simulink model "Regler_fin"  (R2026a)
settings: Solver=ode23s  StartTime=tSim(1)  StopTime=tSim(end)  FixedStep=tStep  EnableMultiTasking=on
values from neighbouring files (symbols this model uses):
  A_grid = zeros(N_ml, 16)    [reglerInit_fin.m]    (also in reglerInit_opt1.m; reglerInit_opt2.m; reglerInit_opt3.m; reglerInit_opt4.m)
  a_ref0 = 0    [reglerInit_fin.m]    (also in reglerInit_opt2.m; reglerInit_opt3.m; reglerInit_opt4.m)
  a_ref_lim = 3.91175    [reglerInit_fin.m]    (also in reglerInit_opt2.m = 3.8; reglerInit_opt3.m = 3.8)
  B = [0; -30.49; 0; 30.49]    [A4_4.m]    (also in reglerInit.m; reglerInit_fin.m; reglerInit_gain_scheduling.m; reglerInit_opt.m)
  C = [1 0 0 0 ... (first row only)    [reglerInit.m]    (also in reglerInit_fin.m; reglerInit_gain_scheduling.m; reglerInit_opt.m; reglerInit_opt1.m)
  d_large = 1.18779    [reglerInit_fin.m]    (also in reglerInit_opt2.m = 1.3; reglerInit_opt3.m = 1.3; reglerInit_opt4.m = 1.2)
  d_small = 0.5719    [reglerInit_fin.m]    (also in reglerInit_opt2.m = 0.45; reglerInit_opt3.m = 0.45; reglerInit_opt4.m = 0.35)
  ff_gain = 0.942931    [reglerInit_fin.m]    (also in reglerInit_opt.m = 1; reglerInit_opt1.m = 1; reglerInit_opt2.m = 1; reglerInit_opt3.m = 1)
  g = 9.81    [reglerInit_fin.m]    (also in reglerInit_opt.m; reglerInit_opt1.m; reglerInit_opt2.m; reglerInit_opt3.m)
  gamma_phi = 0.195386    [reglerInit_fin.m]    (also in reglerInit_opt2.m = 0.3; reglerInit_opt3.m = 0.3; reglerInit_opt4.m = 0)
  j_ref_lim = 24.6332    [reglerInit_fin.m]    (also in reglerInit_opt2.m = 20; reglerInit_opt3.m = 20)
  K_grid = zeros(N_ml, 4)    [reglerInit_fin.m]    (also in reglerInit_opt1.m; reglerInit_opt2.m)
  k_r = 7.2e-3    (= 0.0072)    [reglerInit_fin.m]    (also in reglerInit_opt.m; reglerInit_opt1.m; reglerInit_opt2.m; reglerInit_opt3.m)
  L_grid = zeros(N_ml, 8)    [reglerInit_fin.m]    (also in reglerInit_opt1.m; reglerInit_opt2.m; reglerInit_opt3.m; reglerInit_opt4.m)
  M_ff_max = 0.39    [reglerInit_fin.m]    (also in reglerInit_opt.m = 0.34; reglerInit_opt1.m = 0.34; reglerInit_opt2.m = 0.34; reglerInit_opt3.m = 0.34)
  M_max_total = 0.4    [reglerInit.m]    (also in reglerInit_fin.m; reglerInit_gain_scheduling.m; reglerInit_opt.m; reglerInit_opt1.m)
  m_s = 0.8    [reglerInit_fin.m]    (also in reglerInit_opt.m; reglerInit_opt1.m; reglerInit_opt2.m; reglerInit_opt3.m)
  ml_grid = linspace(1, 5, 17)    [reglerInit_fin.m]    (also in reglerInit_opt1.m; reglerInit_opt2.m; reglerInit_opt3.m; reglerInit_opt4.m)
  omega_ref_large = 2.08014    [reglerInit_fin.m]    (also in reglerInit_opt2.m = 2; reglerInit_opt3.m = 2)
  omega_ref_medium = 3.57058    [reglerInit_fin.m]    (also in reglerInit_opt2.m = 3.3; reglerInit_opt3.m = 3.3)
  omega_ref_small = 3.92272    [reglerInit_fin.m]    (also in reglerInit_opt2.m = 3.3; reglerInit_opt3.m = 3.3)
  phi_ref_lim = deg2rad(35)    [reglerInit_fin.m]    (also in reglerInit_opt2.m = deg2rad(18); reglerInit_opt3.m = deg2rad(18); reglerInit_opt4.m = deg2rad(10))
  phi_slow_1 = deg2rad(26.517)    [reglerInit_fin.m]    (also in reglerInit_opt2.m = deg2rad(28); reglerInit_opt3.m = deg2rad(28); reglerInit_opt4.m = deg2rad(28))
  phi_slow_2 = deg2rad(30.8674)    [reglerInit_fin.m]    (also in reglerInit_opt2.m = deg2rad(36); reglerInit_opt3.m = deg2rad(36); reglerInit_opt4.m = deg2rad(36))
  phidot_ref_lim = 1.6    [reglerInit_fin.m]    (also in reglerInit_opt2.m = 0.8; reglerInit_opt3.m = 0.8; reglerInit_opt4.m = 0)
  r_wheel = 0.041    [reglerInit_fin.m]    (also in reglerInit_opt.m; reglerInit_opt1.m; reglerInit_opt2.m; reglerInit_opt3.m)
  u_max = 100    [reglerInit.m]    (also in reglerInit_fin.m; reglerInit_gain_scheduling.m; reglerInit_opt.m; reglerInit_opt1.m)
  v_ref0 = 0    [reglerInit_fin.m]    (also in reglerInit_opt2.m; reglerInit_opt3.m; reglerInit_opt4.m)
  x_ref0 = 0    [reglerInit_fin.m]    (also in reglerInit_opt2.m; reglerInit_opt3.m; reglerInit_opt4.m)
  xhat0 = [0, 0, 0, 0]    [reglerInit.m]    (also in reglerInit_fin.m = [0; 0; 0; 0]; reglerInit_gain_scheduling.m; reglerInit_opt.m = [0; 0; 0; 0]; reglerInit_opt1.m = [0; 0; 0; 0])
settings Model: Creator=Henning Schlüter  LastModifiedBy=louis
settings DataIOCC: SignalLoggingSaveFormat=ModelDataLogs
settings DebuggingCC: UnderspecifiedInitializationDetection=Classic  PregeneratedLibrarySubsystemCodeDiagnostic=none
settings HardwareCC: ProdHWDeviceType=32-bit Generic
settings GRTTargetCC: CombineOutputUpdateFcns=off  GRTInterface=on

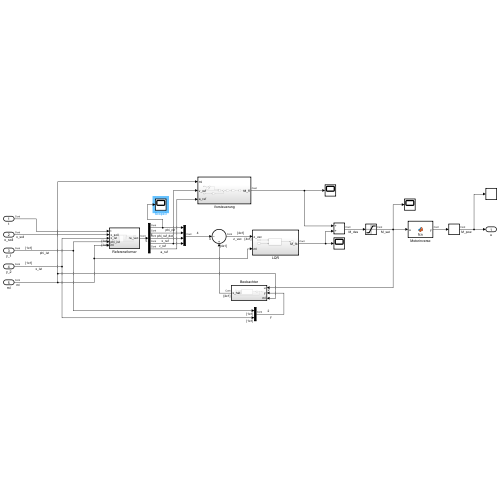
[thumbnail: Simulink's stored preview of the top-level diagram]
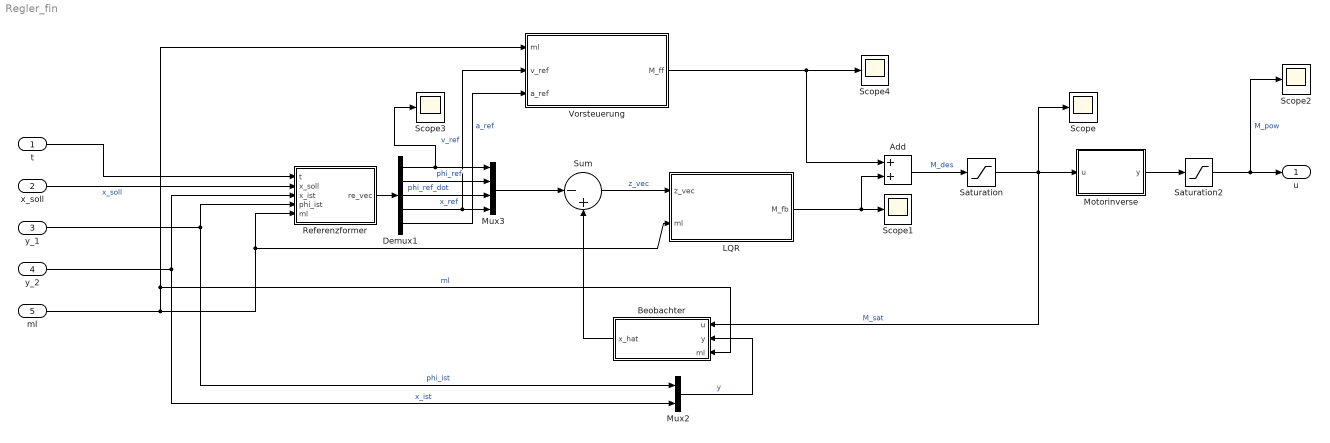
== system Regler_fin ==
  t : Inport  OutDataTypeStr=double  PortDimensions=1  SampleTime=0
  "x_soll " : Inport  Port=2  OutDataTypeStr=double  PortDimensions=1  SampleTime=0
  y_1 : Inport  Port=3  OutDataTypeStr=double  PortDimensions=[1 1]  SampleTime=0
  y_2 : Inport  Port=4  OutDataTypeStr=double  PortDimensions=[1 1]  SampleTime=0
  ml : Inport  Port=5  OutDataTypeStr=double  PortDimensions=1  SampleTime=0
  Add : Sum
  Beobachter : Subsystem
  Demux1 : Demux  Outputs=5
  LQR : Subsystem
  Motorinverse : MATLAB Function  TreatAsAtomicUnit=on
  Mux2 : Mux  Inputs=2
  Mux3 : Mux
  Referenzformer : Subsystem
  Saturation : Saturate  UpperLimit=M_max_total  LowerLimit=-M_max_total
  Saturation2 : Saturate  UpperLimit=u_max  LowerLimit=-u_max  LinearizeAsGain=off
  Scope{,1..4} (5 alike) : Scope
      Scope settings: ActiveDisplayYMinimum=-0.49175375586070769  ActiveDisplayYMaximum=-0.20102751095454277
      Scope1 settings: ActiveDisplayYMinimum=-0.094687281937852363  ActiveDisplayYMaximum=1.6990664417619266
      Scope2 settings: ActiveDisplayYMinimum=27.519723000110169  ActiveDisplayYMaximum=88.458122086201712  DataLoggingVariableName=ScopeData2
      Scope3 settings: ActiveDisplayYMinimum=-0.061908248725805554  ActiveDisplayYMaximum=0.071206311299841979  DataLoggingVariableName=ScopeData3
      Scope4 settings: ActiveDisplayYMinimum=-0.15043823578049448  ActiveDisplayYMaximum=0.16991782466155569  DataLoggingVariableName=ScopeData6
  Sum : Sum  Inputs=|-+
  Vorsteuerung : Subsystem
  u : Outport  OutDataTypeStr=double  PortDimensions=1  VectorParamsAs1DForOutWhenUnconnected=off
  wires:
  Saturation/1 -> Motorinverse/1(u), Beobachter/1(u), Scope/1  "M_sat"
  Motorinverse/1(y) -> Saturation2/1
  Referenzformer/1(re_vec) -> Demux1/1
  y_2/1 -> Mux2/2, Referenzformer/3(x_ist)  "x_ist"
  Saturation2/1 -> u/1, Scope2/1  "M_pow"
  t/1 -> Referenzformer/1(t)
  Mux2/1 -> Beobachter/2(y)  "y"
  "x_soll "/1 -> Referenzformer/2(x_soll)  "x_soll"
  y_1/1 -> Referenzformer/4(phi_ist), Mux2/1  "phi_ist"
  ml/1 -> Beobachter/3(ml), Vorsteuerung/1(ml), LQR/2(ml), Referenzformer/5(ml)  "ml"
  Demux1/1 -> Scope3/1, Mux3/1  "phi_ref"
  Demux1/2 -> Mux3/2  "phi_ref_dot"
  Demux1/3 -> Mux3/3  "x_ref"
  Demux1/4 -> Mux3/4, Vorsteuerung/2(v_ref)  "v_ref"
  Mux3/1 -> Sum/1
  Add/1 -> Saturation/1  "M_des"
  Demux1/5 -> Vorsteuerung/3(a_ref)  "a_ref"
  LQR/1(M_fb) -> Add/2, Scope1/1
  Sum/1 -> LQR/1(z_vec)  "z_vec"
  Beobachter/1(x_hat) -> Sum/2
  Vorsteuerung/1(M_ff) -> Add/1, Scope4/1

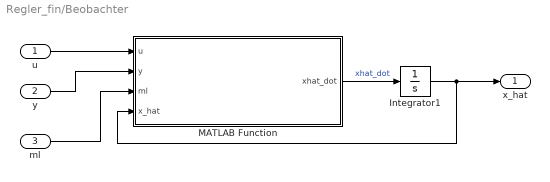
== system Regler_fin/Beobachter ==
  u : Inport
  y : Inport  Port=2
  ml : Inport  Port=3
  Integrator1 : Integrator  InitialCondition=xhat0
  MATLAB Function : MATLAB Function  TreatAsAtomicUnit=on
  x_hat : Outport
  wires:
  u/1 -> MATLAB Function/1(u)
  MATLAB Function/1(xhat_dot) -> Integrator1/1  "xhat_dot"
  Integrator1/1 -> MATLAB Function/4(x_hat), x_hat/1
  ml/1 -> MATLAB Function/3(ml)
  y/1 -> MATLAB Function/2(y)

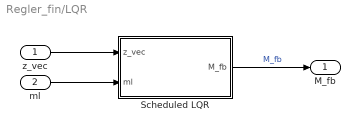
== system Regler_fin/LQR ==
  z_vec : Inport
  ml : Inport  Port=2
  Scheduled LQR : MATLAB Function  TreatAsAtomicUnit=on
  M_fb : Outport
  wires:
  z_vec/1 -> Scheduled LQR/1(z_vec)
  ml/1 -> Scheduled LQR/2(ml)
  Scheduled LQR/1(M_fb) -> M_fb/1  "M_fb"

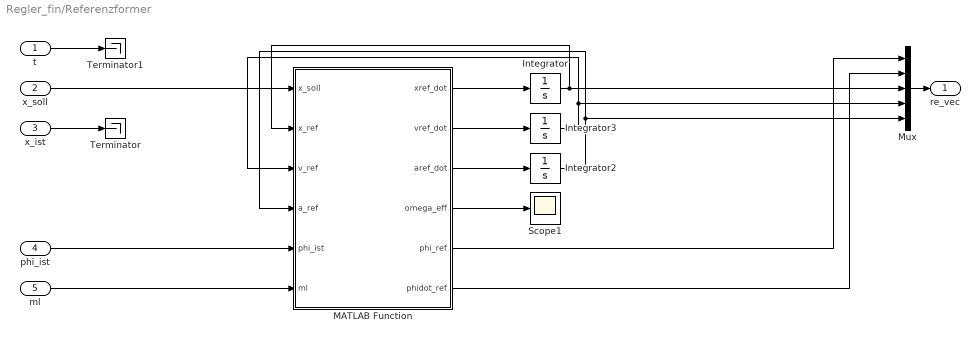
== system Regler_fin/Referenzformer ==
  t : Inport
  x_soll : Inport  Port=2
  x_ist : Inport  Port=3
  phi_ist : Inport  Port=4
  ml : Inport  Port=5
  Integrator : Integrator  InitialCondition=x_ref0
  Integrator2 : Integrator  InitialCondition=a_ref0
  Integrator3 : Integrator  InitialCondition=v_ref0
  MATLAB Function : MATLAB Function  TreatAsAtomicUnit=on
  Mux : Mux  Inputs=5
  Scope1 : Scope
      settings: ActiveDisplayYMinimum=-0.15489744027848928  ActiveDisplayYMaximum=0.17747491637319093  DataLoggingVariableName=ScopeData5
  Terminator : Terminator
  Terminator1 : Terminator
  re_vec : Outport
  wires:
  Mux/1 -> re_vec/1
  t/1 -> Terminator1/1
  phi_ist/1 -> MATLAB Function/5(phi_ist)
  x_ist/1 -> Terminator/1
  ml/1 -> MATLAB Function/6(ml)
  x_soll/1 -> MATLAB Function/1(x_soll)
  MATLAB Function/2(vref_dot) -> Integrator3/1
  MATLAB Function/1(xref_dot) -> Integrator/1
  MATLAB Function/3(aref_dot) -> Integrator2/1
  Integrator/1 -> MATLAB Function/2(x_ref), Mux/3
  Integrator3/1 -> MATLAB Function/3(v_ref), Mux/4
  Integrator2/1 -> MATLAB Function/4(a_ref), Mux/5
  MATLAB Function/6(phidot_ref) -> Mux/2
  MATLAB Function/5(phi_ref) -> Mux/1
  MATLAB Function/4(omega_eff) -> Scope1/1

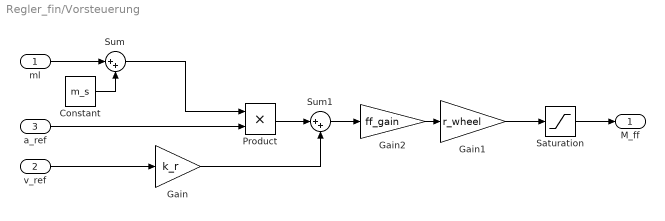
== system Regler_fin/Vorsteuerung ==
  ml : Inport
  v_ref : Inport  Port=2
  a_ref : Inport  Port=3
  Constant : Constant  Value=m_s
  Gain : Gain  Gain=k_r
  Gain1 : Gain  Gain=r_wheel
  Gain2 : Gain  Gain=ff_gain
  Product : Product
  Saturation : Saturate  UpperLimit=M_ff_max  LowerLimit=-M_ff_max
  Sum : Sum  Inputs=|++
  Sum1 : Sum  Inputs=|++
  M_ff : Outport
  wires:
  ml/1 -> Sum/1
  a_ref/1 -> Product/2
  Saturation/1 -> M_ff/1
  v_ref/1 -> Gain/1
  Constant/1 -> Sum/2
  Sum/1 -> Product/1
  Gain1/1 -> Saturation/1
  Gain2/1 -> Gain1/1
  Sum1/1 -> Gain2/1
  Product/1 -> Sum1/1
  Gain/1 -> Sum1/2

== matlab function Regler_fin/Motorinverse ==
  data: u input; y output
function y = fcn(u)

y = sign(u(1)/2)*(9.434*abs(u(1)/2))^2*100/3.56;

== matlab function Regler_fin/LQR/Scheduled LQR ==
  data: z_vec input double size=4; M_fb output double size=1; ml input double size=1; ml_grid parameter double size=17; K_grid parameter double size=[17 4]
function M_fb = ScheduledLQR(z_vec, ml, ml_grid, K_grid)
%#codegen

% Ausgang explizit initialisieren
M_fb = 0.0;

% Eingänge robust lesen
ml = double(ml(1));

z1 = double(z_vec(1));
z2 = double(z_vec(2));
z3 = double(z_vec(3));
z4 = double(z_vec(4));

% ml auf gueltigen Bereich begrenzen
if ml <= ml_grid(1)
    K1 = K_grid(1,1);
    K2 = K_grid(1,2);
    K3 = K_grid(1,3);
    K4 = K_grid(1,4);

elseif ml >= ml_grid(end)
    n = length(ml_grid);
    K1 = K_grid(n,1);
    K2 = K_grid(n,2);
    K3 = K_grid(n,3);
    K4 = K_grid(n,4);

else
    n = length(ml_grid);
    idx = 1;

    for i = 1:n-1
        if ml >= ml_grid(i) && ml <= ml_grid(i+1)
            idx = i;
            break;
        end
    end

    alpha = (ml - ml_grid(idx)) / (ml_grid(idx+1) - ml_grid(idx));

    K1 = (1-alpha)*K_grid(idx,1) + alpha*K_grid(idx+1,1);
    K2 = (1-alpha)*K_grid(idx,2) + alpha*K_grid(idx+1,2);
    K3 = (1-alpha)*K_grid(idx,3) + alpha*K_grid(idx+1,3);
    K4 = (1-alpha)*K_grid(idx,4) + alpha*K_grid(idx+1,4);
end

% LQR Gesetz
M_fb = -(K1*z1 + K2*z2 + K3*z3 + K4*z4);

== matlab function Regler_fin/Beobachter/MATLAB Function ==
  data: u input double size=1; xhat_dot output double size=[4 1]; y input double size=2; ml input double size=1; x_hat input double size=4; ml_grid parameter double size=[1 17]; A_grid parameter double size=[17 16]; L_grid parameter double size=[17 8]; B parameter double size=[4 1]; C parameter double size=[2 4]
function xhat_dot = ScheduledObserver(u, y, ml, x_hat, ml_grid, A_grid, L_grid, B, C)
%#codegen

xhat_dot = zeros(4,1);

% Eingänge robust lesen
u  = double(u(1));
ml = double(ml(1));

y1 = double(y(1));
y2 = double(y(2));

xh1 = double(x_hat(1));
xh2 = double(x_hat(2));
xh3 = double(x_hat(3));
xh4 = double(x_hat(4));

% Scheduling-Index und Interpolation
if ml <= ml_grid(1)
    idx = 1;
    alpha = 0.0;

elseif ml >= ml_grid(end)
    idx = length(ml_grid) - 1;
    alpha = 1.0;

else
    n = length(ml_grid);
    idx = 1;

    for i = 1:n-1
        if ml >= ml_grid(i) && ml <= ml_grid(i+1)
            idx = i;
            break;
        end
    end

    alpha = (ml - ml_grid(idx)) / (ml_grid(idx+1) - ml_grid(idx));
end

% A und L interpolieren
Arow = zeros(1,16);
Lrow = zeros(1,8);

for j = 1:16
    Arow(j) = (1-alpha)*A_grid(idx,j) + alpha*A_grid(idx+1,j);
end

for j = 1:8
    Lrow(j) = (1-alpha)*L_grid(idx,j) + alpha*L_grid(idx+1,j);
end

A_ml = reshape(Arow, 4, 4);
L_ml = reshape(Lrow, 4, 2);

xv = [xh1; xh2; xh3; xh4];
yv = [y1; y2];


y_hat = C * xv;
e_y = yv - y_hat;

xhat_dot = A_ml*xv + B*u + L_ml*e_y;

== matlab function Regler_fin/Referenzformer/MATLAB Function ==
  data: x_soll input double size=1; xref_dot output double size=1; x_ref input double size=1; v_ref input double size=1; a_ref input double size=1; phi_ist input double size=1; ml input double size=1; vref_dot output double size=1; aref_dot output double size=1; omega_eff output double size=1; phi_ref output double size=1; phidot_ref_lim parameter double size=[1 1]; g parameter double size=[1 1]; gamma_phi parameter double size=[1 1]; phi_ref_lim parameter double size=[1 1]; j_ref_lim parameter double size=[1 1]; a_ref_lim parameter double size=[1 1]; phi_slow_2 parameter double size=[1 1]; phi_slow_1 parameter double size=[1 1]; d_small parameter double size=[1 1]; d_large parameter double size=[1 1]; omega_ref_small parameter double size=[1 1]; omega_ref_medium parameter double size=[1 1]; omega_ref_large parameter double size=[1 1]; phidot_ref output double size=1
function [xref_dot, vref_dot, aref_dot, omega_eff, phi_ref, phidot_ref] = AdaptiveTrajDyn(x_soll, x_ref, v_ref, a_ref, phi_ist, ml, phidot_ref_lim, g, gamma_phi, phi_ref_lim, j_ref_lim, a_ref_lim, phi_slow_2, phi_slow_1, d_small, d_large, omega_ref_small, omega_ref_medium, omega_ref_large)
%#codegen

% Eingänge robust als Skalare lesen
x_soll  = double(x_soll(1));
x_ref   = double(x_ref(1));
v_ref   = double(v_ref(1));
a_ref   = double(a_ref(1));
phi_ist = double(phi_ist(1));
ml      = double(ml(1));

% Outputs explizit initialisieren
xref_dot   = 0.0;
vref_dot   = 0.0;
aref_dot   = 0.0;
omega_eff  = 0.0;
phi_ref    = 0.0;
phidot_ref = 0.0;

% Abstand zwischen interner Referenz und Soll
d = abs(x_soll - x_ref);

% Adaptive Wahl von omega
if d > d_large
    omega_eff = omega_ref_large;
elseif d > d_small
    omega_eff = omega_ref_medium;
else
    omega_eff = omega_ref_small;
end

% Massenabhängige leichte Anpassung
if ml > 4.0
    omega_eff = 0.90 * omega_eff;
elseif ml < 1.5
    omega_eff = 1.05 * omega_eff;
end

% Sicherheitsreduktion bei großem Pendelausschlag
phi_abs = abs(phi_ist);

if phi_abs > phi_slow_2
    omega_eff = 0.55 * omega_eff;
elseif phi_abs > phi_slow_1
    omega_eff = 0.75 * omega_eff;
end

% Schutz gegen numerisch unguenstige Werte
if omega_eff < 0.2
    omega_eff = 0.2;
elseif omega_eff > 8.0
    omega_eff = 8.0;
end

% Kontinuierlicher Filter 3. Ordnung:
% x''' = omega^3*(x_soll-x_ref) - 3*omega^2*v_ref - 3*omega*a_ref
j_cmd = omega_eff * omega_eff * omega_eff * (x_soll - x_ref) ...
      - 3.0 * omega_eff * omega_eff * v_ref ...
      - 3.0 * omega_eff * a_ref;



% Massenabhaengige Jerk-Grenze
j_eff_lim = j_ref_lim;

if ml > 4.0
    j_eff_lim = 0.55 * j_eff_lim;
elseif ml > 3.0
    j_eff_lim = 0.70 * j_eff_lim;
elseif ml > 2.0
    j_eff_lim = 0.85 * j_eff_lim;
end

% Jerk-Begrenzung
if j_cmd > j_eff_lim
    j_cmd = j_eff_lim;
elseif j_cmd < -j_eff_lim
    j_cmd = -j_eff_lim;
end


% Massenabhaengige Beschleunigungsgrenze
a_eff_lim = a_ref_lim;

if ml > 4.0
    a_eff_lim = min(a_eff_lim, 1.55);
elseif ml > 3.0
    a_eff_lim = min(a_eff_lim, 2.10);
elseif ml > 2.0
    a_eff_lim = min(a_eff_lim, 2.80);
end

% Beschleunigungsbegrenzung
if a_ref > a_eff_lim && j_cmd > 0.0
    j_cmd = 0.0;
elseif a_ref < -a_eff_lim && j_cmd < 0.0
    j_cmd = 0.0;
end

% Integratordynamik
xref_dot = v_ref;
vref_dot = a_ref;
aref_dot = j_cmd;

% Partielle Pendelreferenz
phi_ref = gamma_phi * (-a_ref / g);

if phi_ref > phi_ref_lim
    phi_ref = phi_ref_lim;
elseif phi_ref < -phi_ref_lim
    phi_ref = -phi_ref_lim;
end


phidot_ref = gamma_phi * (-j_cmd / g);

if phidot_ref > phidot_ref_lim
    phidot_ref = phidot_ref_lim;
elseif phidot_ref < -phidot_ref_lim
    phidot_ref = -phidot_ref_lim;
end
